simulink model "CSTFM_Pclass"  (Simulink 8.5)
settings: Solver=ode1  SolverMode=SingleTasking  StartTime=0.0  StopTime=200  FixedStep=25e-6  RelTol=1e-3
libraries: dspswit3 x1
settings Model: Creator=Administrator  LastModifiedBy=Administrator
settings DataIOCC: SignalLoggingSaveFormat=Dataset  SaveOutput=off  SaveTime=off
settings OptimizationCC: BlockReduction=off  OptimizeBlockIOStorage=off  BufferReuse=off  GlobalBufferReuse=off  ExpressionFolding=off  ExpressionDepthLimit=128  LocalBlockOutputs=off
settings DebuggingCC: UnderspecifiedInitializationDetection=Simplified  MergeDetectMultiDrivingBlocksExec=error  FcnCallInpInsideContextMsg=EnableAllAsError  StateNameClashWarn=none
settings GRTTargetCC: CombineOutputUpdateFcns=on  GRTInterface=off

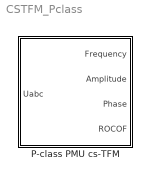
== system CSTFM_Pclass ==
  P-class PMU cs-TFM : Subsystem  SystemSampleTime=2e-4  VariantControl=variant3  mask{nominal_freq=50, T=0.06, Fs=5e3, Fr_50=50}
      mask prompts: nominal_freq "Norminal Frequency"; T "Window length (s)"; Fs "Sampling rate (Hz)"; Fr_50 "Data report rate (frames/s)"
      mask init:
      | %% // PUM initialization//
      | % the file is used to set basic paramters and creat initial matrix  
      | 
      | %% basic paramters
      | nominal_freq = 50;
      | T=0.06; %0.1;
      | TdF=10;
      | data_rate_50=1; %case: 1(10),2(25),3(50)
      | Fs=5e3;
      | P=11;
      | 
      | %% creat intial matrix
      | f0 = nominal_freq;
      | 
      | switch data_rate_50
      | case 1
      | Fr_50 = 10;
      | case 2
      | Fr_50 = 25;
      | case 3
      | Fr_50 = 50;
      | otherwise
      | display('Non contemplated data reporting rate')
      | end
      | 
      | Ts=1/Fs;
      | dF = 1/T;
      | M = round(T*Fs);
      | overlap=2*M/3;
      | kmax = round(f0*T);
      | k = (kmax-2):(kmax+7);
      | Wk = exp(-1i*2*pi*k./M);
      | NumIters=2;
      | Fr = Fr_50;
      | Tr = 1/Fr;
      | H = M*P;
      | 
      | h_axis = 0:Fs/H:Fs*(H-1)/H; % matrix h_aixs
      | 
      | D = zeros(M,H);%
      | for k = 0:M-1
      |     for h = 0:H-1
      |     esp = k - M*h/H;
      |     esp = esp*(M-1)/M;
      |     a = pi*(k-(h/H)*M);
      |     b = a/M;
      |     if b == pi || b == 0
      |         s = 1;
      |     else
      |         s = sin(a)/(M*sin(b));
      |     end
      |     D(k+1,h+1) = s*exp(-1i*pi*esp);
      |     end
      | end
      | 
      | D_funda=D(2:10, 31:37);%D(2:17,51:61);%
      | D_funda=D_funda'; 
      | inter_index=[8,11,14,17,51,54,57,60];%[12 17 23 28 83 89 94 100];
      | D_inter=D(2:10,inter_index);%D(2:17,inter_index);
      | D_inter=D_inter';
      | f_fund=h_axis(31:37);%h_axis(51:61);
      | % dft_rec=zeros(11,16);
      | % freq=(10:10:160);
      | % 
      | % for i=1:11
      | %     ff0=f_fund(i);
      | %     dft_rec(i,:) =(0.5*sinc((freq-ff0)*T)+0.25*sinc((freq-ff0-1/T)*T)+0.25*sinc((freq-ff0+1/T)*T))...
      | %     +  (0.5*sinc((-freq+ff0)*T)+0.25*sinc((-freq+ff0-1/T)*T)+0.25*sinc((-freq+ff0+1/T)*T));
      | % end
      | 
      | order = 2;
      | % M=3*M/5;
      | matrix_f=zeros(M,6,11);%
      | h=1;
      | Nh=M/2;
      | freq=(45:1:55);
      | for index=1:11
      |     omega1=2*pi*freq(index)/Fs;
      |     for i=0:M-1
      |         n = i - Nh;
      |         nc = 0;
      |         facts = factorial(2:-1:0);
      |         e = exp(1j*n*h*omega1);
      |         matrix_f(i+1,nc+1:nc+2*order+2,index) = [(((n*Ts).^...
      |             (order:-1:0)).*e)./facts, (((n*Ts).^...
      |             (0:1:order)).*e')./fliplr(facts)];
      |     end
      | end
      | 
      | matrix_har2=zeros(M,6,11); %
      | freq=2*(45:1:55);
      | for index=1:11
      |     omega1=2*pi*freq(index)/Fs;
      |     for i=0:M-1
      |         n = i - Nh;
      |         nc = 0;
      |         facts = factorial(2:-1:0);
      |         e = exp(1j*n*h*omega1);
      |         matrix_har2(i+1,nc+1:nc+2*order+2,index) = [(((n*Ts).^...
      |             (order:-1:0)).*e)./facts, (((n*Ts).^...
      |             (0:1:order)).*e')./fliplr(facts)];
      |     end
      | end
      | 
      | matrix_har3=zeros(M,6,11);%
      | freq=3*(45:1:55);
      | for index=1:11
      |     omega1=2*pi*freq(index)/Fs;
      |     for i=0:M-1
      |         n = i - Nh;
      |         nc = 0;
      |         facts = factorial(2:-1:0);
      |         e = exp(1j*n*h*omega1);
      |         matrix_har3(i+1,nc+1:nc+2*order+2,index) = [(((n*Ts).^...
      |             (order:-1:0)).*e)./facts, (((n*Ts).^...
      |             (0:1:order)).*e')./fliplr(facts)];
      |     end
      | end
      | 
      | % M = round(T*Fs);
      | clear D
      mask TypeOptions Fr_50: 10 | 25 | 50

== system CSTFM_Pclass/P-class PMU cs-TFM ==
  Uabc : Inport
  Buffer : Buffer  N=M  V=overlap  TreatMby1Signals=One channel
  Demux : Demux  Outputs=3
  Rate Transition : RateTransition  OutPortSampleTime=2e-4
  Subsystem : Subsystem  TreatAsAtomicUnit=on  SystemSampleTime=Ts*(M-overlap)
  Terminator : Terminator
  Terminator1 : Terminator
  msdft Hanning : Subsystem  TreatAsAtomicUnit=on  SystemSampleTime=2e-4
  Frequency : Outport
  Amplitude : Outport  Port=2
  Phase : Outport  Port=3
  ROCOF : Outport  Port=4
  wires:
  Uabc/1 -> Demux/1
  Rate Transition/1 -> Buffer/1
  msdft Hanning/1(DFT) -> Subsystem/2(A)
  Subsystem/4(RoCoF) -> ROCOF/1
  Subsystem/3(frequency) -> Frequency/1
  Subsystem/2(phase_estimated) -> Phase/1
  Subsystem/1(Amplitude) -> Amplitude/1
  Buffer/1 -> Subsystem/1(buffer_a)
  Demux/3 -> Terminator1/1
  Demux/2 -> Terminator/1
  Demux/1 -> msdft Hanning/1(signal), Rate Transition/1  "Ua"

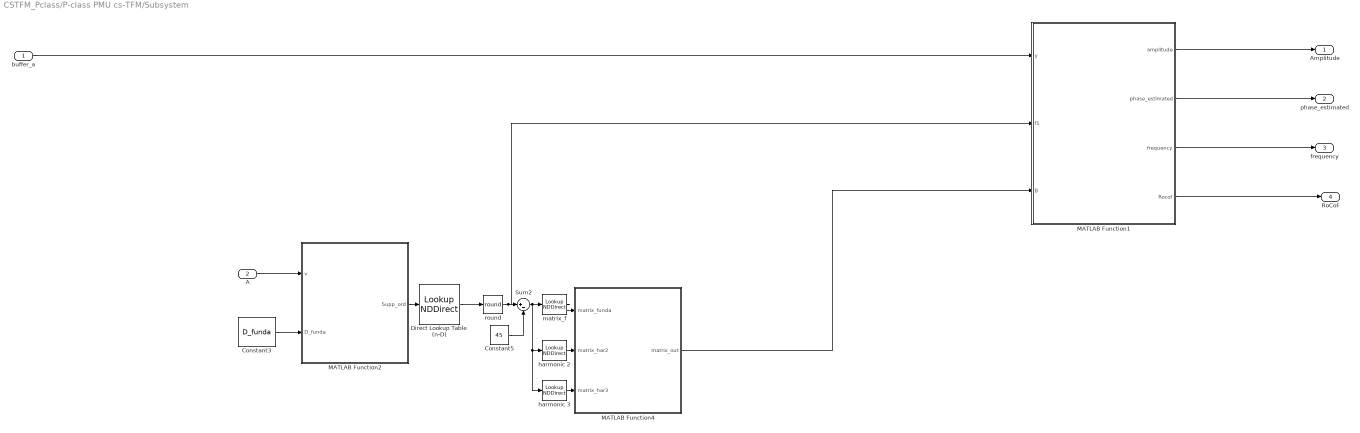
== system CSTFM_Pclass/P-class PMU cs-TFM/Subsystem ==
  buffer_a : Inport
  A : Inport  Port=2
  Constant3 : Constant  Value=D_funda
  Constant5 : Constant  Value=45
  Direct Lookup Table (n-D) : LookupNDDirect  NumberOfTableDimensions=1  Table=h_axis
  MATLAB Function1 : MATLAB Function  RequirementInfo={} %GIDa_f55fb0f0_c66f_4964_a101_9f74e0196493  SystemSampleTime=Ts*(M-overlap)
  MATLAB Function2 : MATLAB Function  SystemSampleTime=Ts*(M-overlap)
  MATLAB Function4 : MATLAB Function  RequirementInfo={} %GIDa_9de8f8bb_0410_4add_86be_2b397df83b55  SystemSampleTime=Ts*(M-overlap)
  Sum2 : Sum  Inputs=|+-
  harmonic 2 : LookupNDDirect  NumberOfTableDimensions=3  InputsSelectThisObjectFromTable=2-D Matrix  Table=matrix_har2
  "harmonic 3 " : LookupNDDirect  NumberOfTableDimensions=3  InputsSelectThisObjectFromTable=2-D Matrix  Table=matrix_har3
  matrix_f : LookupNDDirect  NumberOfTableDimensions=3  InputsSelectThisObjectFromTable=2-D Matrix  Table=matrix_f
  round : Rounding  Operator=round
  Amplitude : Outport
  phase_estimated : Outport  Port=2
  frequency : Outport  Port=3
  RoCoF : Outport  Port=4
  wires:
  Direct Lookup Table (n-D)/1 -> round/1
  MATLAB Function1/4(Rocof) -> RoCoF/1
  buffer_a/1 -> MATLAB Function1/1(y)
  round/1 -> Sum2/1, MATLAB Function1/2(f1)
  Constant3/1 -> MATLAB Function2/2(D_funda)
  MATLAB Function2/1(Supp_ord) -> Direct Lookup Table (n-D)/1
  A/1 -> MATLAB Function2/1(v)
  matrix_f/1 -> MATLAB Function4/1(matrix_funda)
  Sum2/1 -> "harmonic 3 "/1, harmonic 2/1, matrix_f/1
  Constant5/1 -> Sum2/2
  harmonic 2/1 -> MATLAB Function4/2(matrix_har2)
  "harmonic 3 "/1 -> MATLAB Function4/3(matrix_har3)
  MATLAB Function4/1(matrix_out) -> MATLAB Function1/3(B)
  MATLAB Function1/1(amplitude) -> Amplitude/1
  MATLAB Function1/2(phase_estimated) -> phase_estimated/1
  MATLAB Function1/3(frequency) -> frequency/1

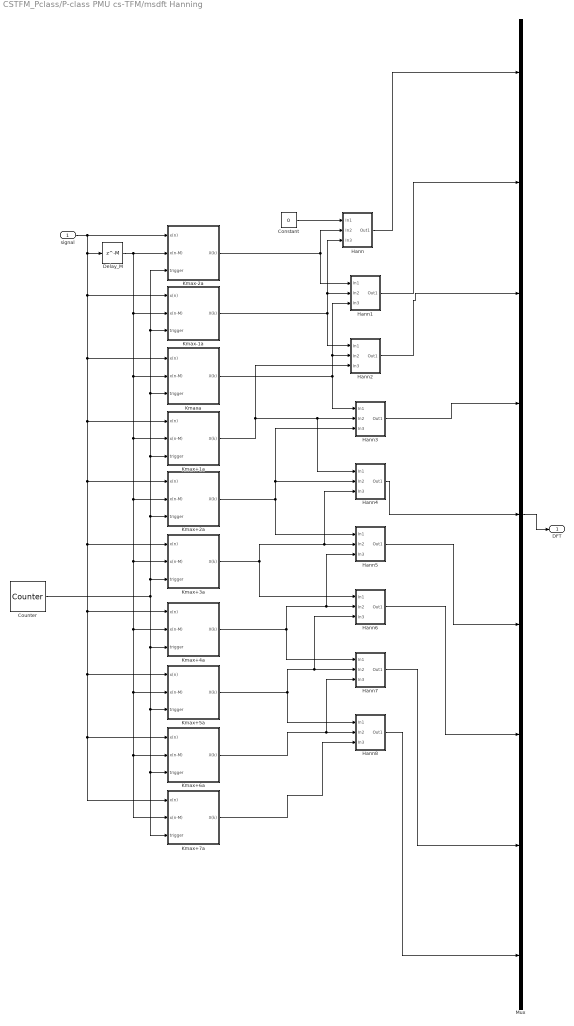
== system CSTFM_Pclass/P-class PMU cs-TFM/msdft Hanning ==
  signal : Inport
  Constant : Constant  Value=0
  Counter : dspswit3/Counter  Direction=Up  CountEvent=Free running  CounterSize=User defined  MaxCount=M-1  InitialCount=1  Output=Hit  HitValue=0  ResetInput=off  SamplesPerFrame=1  Ts=Ts  CntDtype=double  HitDtype=Logical
  Delay_M : Delay  DelayLength=M
  Hann : Subsystem
  Hann1 : Subsystem
  Hann2 : Subsystem
  Hann3 : Subsystem
  Hann4 : Subsystem
  Hann5 : Subsystem
  Hann6 : Subsystem
  Hann7 : Subsystem
  Hann8 : Subsystem
  Kmax+1a : Subsystem
  Kmax+2a : Subsystem
  Kmax+3a : Subsystem
  Kmax+4a : Subsystem
  Kmax+5a : Subsystem
  Kmax+6a : Subsystem
  Kmax+7a : Subsystem
  Kmax-1a : Subsystem
  Kmax-2a : Subsystem
  Kmaxa : Subsystem
  Mux : Mux  Inputs=9
  DFT : Outport
  wires:
  Counter/1 -> Kmax+5a/3(trigger), Kmax+7a/3(trigger), Kmax+6a/3(trigger), Kmax+4a/3(trigger), Kmax+2a/3(trigger), Kmax+1a/3(trigger), Kmax-1a/3(trigger), Kmax-2a/3(trigger), Kmaxa/3(trigger), Kmax+3a/3(trigger)
  Kmax-2a/1(X(k)) -> Hann/2(In2), Hann1/1(In1)
  Kmax-1a/1(X(k)) -> Hann2/1(In1), Hann1/2(In2), Hann/3(In3)
  Kmaxa/1(X(k)) -> Hann3/1(In1), Hann2/2(In2), Hann1/3(In3)
  Kmax+1a/1(X(k)) -> Hann2/3(In3), Hann4/1(In1), Hann3/2(In2)
  Kmax+2a/1(X(k)) -> Hann4/2(In2), Hann3/3(In3), Hann5/1(In1)
  Kmax+4a/1(X(k)) -> Hann7/1(In1), Hann5/3(In3), Hann6/2(In2)
  Kmax+6a/1(X(k)) -> Hann7/3(In3), Hann8/2(In2)
  Mux/1 -> DFT/1
  signal/1 -> Kmax+7a/1(x(n)), Kmax+6a/1(x(n)), Kmax+5a/1(x(n)), Kmax+4a/1(x(n)), Kmax+3a/1(x(n)), Kmax+2a/1(x(n)), Kmax+1a/1(x(n)), Kmaxa/1(x(n)), Kmax-1a/1(x(n)), Delay_M/1, Kmax-2a/1(x(n))
  Delay_M/1 -> Kmax+5a/2(x(n-M)), Kmax+7a/2(x(n-M)), Kmax+6a/2(x(n-M)), Kmax+4a/2(x(n-M)), Kmax+3a/2(x(n-M)), Kmax+2a/2(x(n-M)), Kmax+1a/2(x(n-M)), Kmaxa/2(x(n-M)), Kmax-1a/2(x(n-M)), Kmax-2a/2(x(n-M))
  Hann/1(Out1) -> Mux/1
  Constant/1 -> Hann/1(In1)
  Hann1/1(Out1) -> Mux/2
  Hann2/1(Out1) -> Mux/3
  Hann3/1(Out1) -> Mux/4
  Hann4/1(Out1) -> Mux/5
  Hann5/1(Out1) -> Mux/6
  Hann6/1(Out1) -> Mux/7
  Hann7/1(Out1) -> Mux/8
  Hann8/1(Out1) -> Mux/9
  Kmax+7a/1(X(k)) -> Hann8/3(In3)
  Kmax+5a/1(X(k)) -> Hann8/1(In1), Hann6/3(In3), Hann7/2(In2)
  Kmax+3a/1(X(k)) -> Hann4/3(In3), Hann5/2(In2), Hann6/1(In1)

== system CSTFM_Pclass/P-class PMU cs-TFM/msdft Hanning/Hann ==
  In1 : Inport
  In2 : Inport  Port=2
  In3 : Inport  Port=3
  Gain : Gain  Gain=-0.25
  Gain1 : Gain  Gain=0.5
  Gain2 : Gain  Gain=-0.25
  Sum : Sum  Inputs=|+++
  Out1 : Outport
  wires:
  Sum/1 -> Out1/1
  In3/1 -> Gain2/1
  In1/1 -> Gain/1
  In2/1 -> Gain1/1
  Gain2/1 -> Sum/3
  Gain1/1 -> Sum/2
  Gain/1 -> Sum/1

== system CSTFM_Pclass/P-class PMU cs-TFM/msdft Hanning/Hann1 ==
  In1 : Inport
  In2 : Inport  Port=2
  In3 : Inport  Port=3
  Gain : Gain  Gain=-0.25
  Gain1 : Gain  Gain=0.5
  Gain2 : Gain  Gain=-0.25
  Sum : Sum  Inputs=|+++
  Out1 : Outport
  wires:
  Sum/1 -> Out1/1
  In3/1 -> Gain2/1
  In1/1 -> Gain/1
  In2/1 -> Gain1/1
  Gain2/1 -> Sum/3
  Gain1/1 -> Sum/2
  Gain/1 -> Sum/1

== system CSTFM_Pclass/P-class PMU cs-TFM/msdft Hanning/Hann2 ==
  In1 : Inport
  In2 : Inport  Port=2
  In3 : Inport  Port=3
  Gain : Gain  Gain=-0.25
  Gain1 : Gain  Gain=0.5
  Gain2 : Gain  Gain=-0.25
  Sum : Sum  Inputs=|+++
  Out1 : Outport
  wires:
  Sum/1 -> Out1/1
  In3/1 -> Gain2/1
  In1/1 -> Gain/1
  In2/1 -> Gain1/1
  Gain2/1 -> Sum/3
  Gain1/1 -> Sum/2
  Gain/1 -> Sum/1

== system CSTFM_Pclass/P-class PMU cs-TFM/msdft Hanning/Hann3 ==
  In1 : Inport
  In2 : Inport  Port=2
  In3 : Inport  Port=3
  Gain : Gain  Gain=-0.25
  Gain1 : Gain  Gain=0.5
  Gain2 : Gain  Gain=-0.25
  Sum : Sum  Inputs=|+++
  Out1 : Outport
  wires:
  Sum/1 -> Out1/1
  In3/1 -> Gain2/1
  In1/1 -> Gain/1
  In2/1 -> Gain1/1
  Gain2/1 -> Sum/3
  Gain1/1 -> Sum/2
  Gain/1 -> Sum/1

== system CSTFM_Pclass/P-class PMU cs-TFM/msdft Hanning/Hann4 ==
  In1 : Inport
  In2 : Inport  Port=2
  In3 : Inport  Port=3
  Gain : Gain  Gain=-0.25
  Gain1 : Gain  Gain=0.5
  Gain2 : Gain  Gain=-0.25
  Sum : Sum  Inputs=|+++
  Out1 : Outport
  wires:
  Sum/1 -> Out1/1
  In3/1 -> Gain2/1
  In1/1 -> Gain/1
  In2/1 -> Gain1/1
  Gain2/1 -> Sum/3
  Gain1/1 -> Sum/2
  Gain/1 -> Sum/1

== system CSTFM_Pclass/P-class PMU cs-TFM/msdft Hanning/Hann5 ==
  In1 : Inport
  In2 : Inport  Port=2
  In3 : Inport  Port=3
  Gain : Gain  Gain=-0.25
  Gain1 : Gain  Gain=0.5
  Gain2 : Gain  Gain=-0.25
  Sum : Sum  Inputs=|+++
  Out1 : Outport
  wires:
  Sum/1 -> Out1/1
  In3/1 -> Gain2/1
  In1/1 -> Gain/1
  In2/1 -> Gain1/1
  Gain2/1 -> Sum/3
  Gain1/1 -> Sum/2
  Gain/1 -> Sum/1

== system CSTFM_Pclass/P-class PMU cs-TFM/msdft Hanning/Hann6 ==
  In1 : Inport
  In2 : Inport  Port=2
  In3 : Inport  Port=3
  Gain : Gain  Gain=-0.25
  Gain1 : Gain  Gain=0.5
  Gain2 : Gain  Gain=-0.25
  Sum : Sum  Inputs=|+++
  Out1 : Outport
  wires:
  Sum/1 -> Out1/1
  In3/1 -> Gain2/1
  In1/1 -> Gain/1
  In2/1 -> Gain1/1
  Gain2/1 -> Sum/3
  Gain1/1 -> Sum/2
  Gain/1 -> Sum/1

== system CSTFM_Pclass/P-class PMU cs-TFM/msdft Hanning/Hann7 ==
  In1 : Inport
  In2 : Inport  Port=2
  In3 : Inport  Port=3
  Gain : Gain  Gain=-0.25
  Gain1 : Gain  Gain=0.5
  Gain2 : Gain  Gain=-0.25
  Sum : Sum  Inputs=|+++
  Out1 : Outport
  wires:
  Sum/1 -> Out1/1
  In3/1 -> Gain2/1
  In1/1 -> Gain/1
  In2/1 -> Gain1/1
  Gain2/1 -> Sum/3
  Gain1/1 -> Sum/2
  Gain/1 -> Sum/1

== system CSTFM_Pclass/P-class PMU cs-TFM/msdft Hanning/Hann8 ==
  In1 : Inport
  In2 : Inport  Port=2
  In3 : Inport  Port=3
  Gain : Gain  Gain=-0.25
  Gain1 : Gain  Gain=0.5
  Gain2 : Gain  Gain=-0.25
  Sum : Sum  Inputs=|+++
  Out1 : Outport
  wires:
  Sum/1 -> Out1/1
  In3/1 -> Gain2/1
  In1/1 -> Gain/1
  In2/1 -> Gain1/1
  Gain2/1 -> Sum/3
  Gain1/1 -> Sum/2
  Gain/1 -> Sum/1

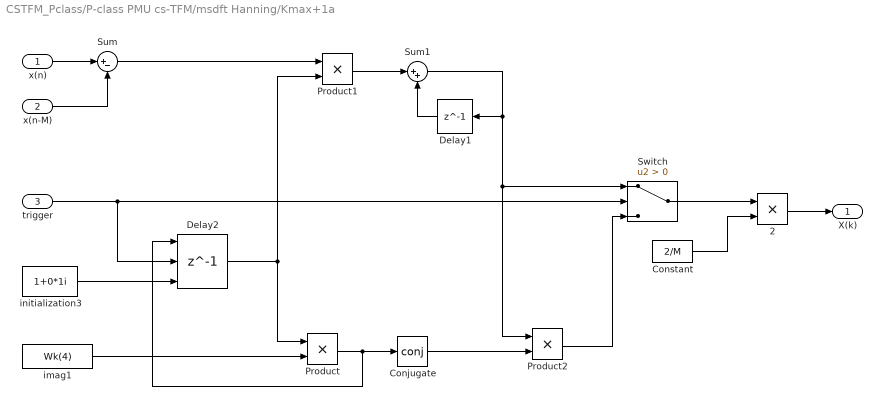
== system CSTFM_Pclass/P-class PMU cs-TFM/msdft Hanning/Kmax+1a ==
  x(n) : Inport
  x(n-M) : Inport  Port=2
  trigger : Inport  Port=3
  2 : Product  RndMeth=Zero
  Conjugate : Math  Operator=conj  SaturateOnIntegerOverflow=on
  Constant : Constant  Value=2/M
  Delay1 : Delay  DelayLength=1
  Delay2 : Delay  DelayLength=1  InitialConditionSource=Input port  ExternalReset=Falling
      settings: InputPortMap=u0,r5,p4
  Product : Product  RndMeth=Zero
  Product1 : Product  RndMeth=Zero
  Product2 : Product  RndMeth=Zero
  Sum : Sum  Inputs=|+-
  Sum1 : Sum  Inputs=|++
  Switch : Switch  Criteria=u2 > Threshold
  imag1 : Constant  Value=Wk(4)
  initialization3 : Constant  Value=1+0*1i
  X(k) : Outport
  wires:
  Switch/1 -> 2/1
  Product2/1 -> Switch/3
  Conjugate/1 -> Product2/2
  Product/1 -> Conjugate/1, Delay2/1
  imag1/1 -> Product/2
  initialization3/1 -> Delay2/3
  Delay2/1 -> Product/1, Product1/2
  trigger/1 -> Switch/2, Delay2/2
  2/1 -> X(k)/1
  Constant/1 -> 2/2
  Sum/1 -> Product1/1
  x(n-M)/1 -> Sum/2
  x(n)/1 -> Sum/1
  Delay1/1 -> Sum1/2
  Sum1/1 -> Product2/1, Switch/1, Delay1/1
  Product1/1 -> Sum1/1

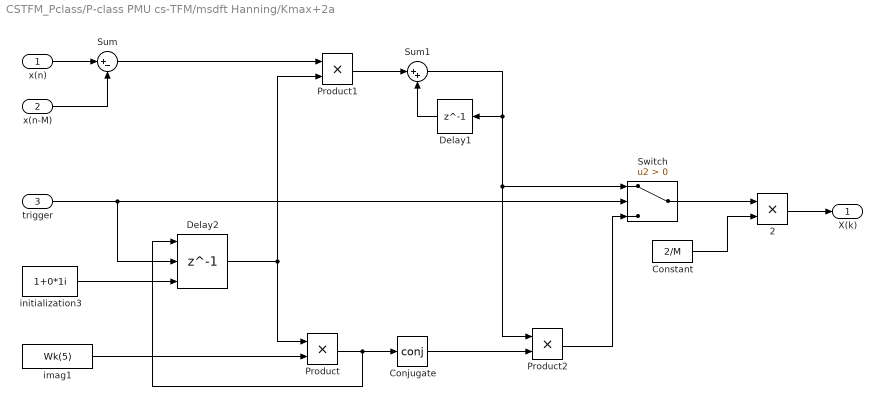
== system CSTFM_Pclass/P-class PMU cs-TFM/msdft Hanning/Kmax+2a ==
  x(n) : Inport
  x(n-M) : Inport  Port=2
  trigger : Inport  Port=3
  2 : Product  RndMeth=Zero
  Conjugate : Math  Operator=conj  SaturateOnIntegerOverflow=on
  Constant : Constant  Value=2/M
  Delay1 : Delay  DelayLength=1
  Delay2 : Delay  DelayLength=1  InitialConditionSource=Input port  ExternalReset=Falling
      settings: InputPortMap=u0,r5,p4
  Product : Product  RndMeth=Zero
  Product1 : Product  RndMeth=Zero
  Product2 : Product  RndMeth=Zero
  Sum : Sum  Inputs=|+-
  Sum1 : Sum  Inputs=|++
  Switch : Switch  Criteria=u2 > Threshold
  imag1 : Constant  Value=Wk(5)
  initialization3 : Constant  Value=1+0*1i
  X(k) : Outport
  wires:
  Switch/1 -> 2/1
  Product2/1 -> Switch/3
  Conjugate/1 -> Product2/2
  Product/1 -> Conjugate/1, Delay2/1
  imag1/1 -> Product/2
  initialization3/1 -> Delay2/3
  Delay2/1 -> Product/1, Product1/2
  trigger/1 -> Switch/2, Delay2/2
  2/1 -> X(k)/1
  Constant/1 -> 2/2
  Sum/1 -> Product1/1
  x(n-M)/1 -> Sum/2
  x(n)/1 -> Sum/1
  Delay1/1 -> Sum1/2
  Sum1/1 -> Product2/1, Switch/1, Delay1/1
  Product1/1 -> Sum1/1

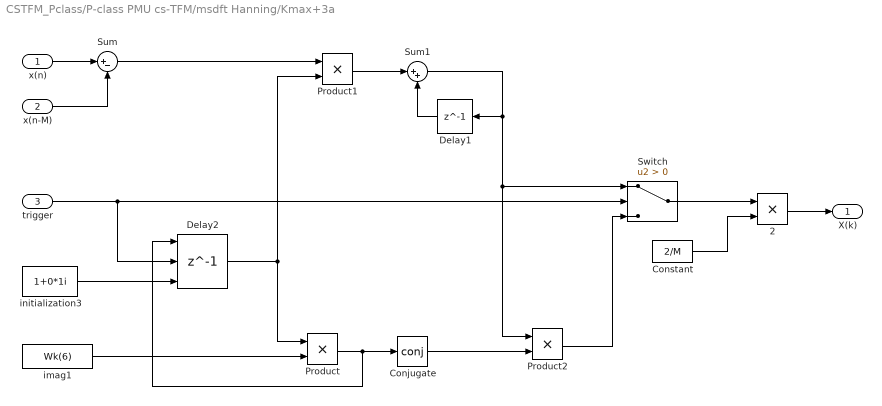
== system CSTFM_Pclass/P-class PMU cs-TFM/msdft Hanning/Kmax+3a ==
  x(n) : Inport
  x(n-M) : Inport  Port=2
  trigger : Inport  Port=3
  2 : Product  RndMeth=Zero
  Conjugate : Math  Operator=conj  SaturateOnIntegerOverflow=on
  Constant : Constant  Value=2/M
  Delay1 : Delay  DelayLength=1
  Delay2 : Delay  DelayLength=1  InitialConditionSource=Input port  ExternalReset=Falling
      settings: InputPortMap=u0,r5,p4
  Product : Product  RndMeth=Zero
  Product1 : Product  RndMeth=Zero
  Product2 : Product  RndMeth=Zero
  Sum : Sum  Inputs=|+-
  Sum1 : Sum  Inputs=|++
  Switch : Switch  Criteria=u2 > Threshold
  imag1 : Constant  Value=Wk(6)
  initialization3 : Constant  Value=1+0*1i
  X(k) : Outport
  wires:
  Switch/1 -> 2/1
  Product2/1 -> Switch/3
  Conjugate/1 -> Product2/2
  Product/1 -> Conjugate/1, Delay2/1
  imag1/1 -> Product/2
  initialization3/1 -> Delay2/3
  Delay2/1 -> Product/1, Product1/2
  trigger/1 -> Switch/2, Delay2/2
  2/1 -> X(k)/1
  Constant/1 -> 2/2
  Sum/1 -> Product1/1
  x(n-M)/1 -> Sum/2
  x(n)/1 -> Sum/1
  Delay1/1 -> Sum1/2
  Sum1/1 -> Product2/1, Switch/1, Delay1/1
  Product1/1 -> Sum1/1

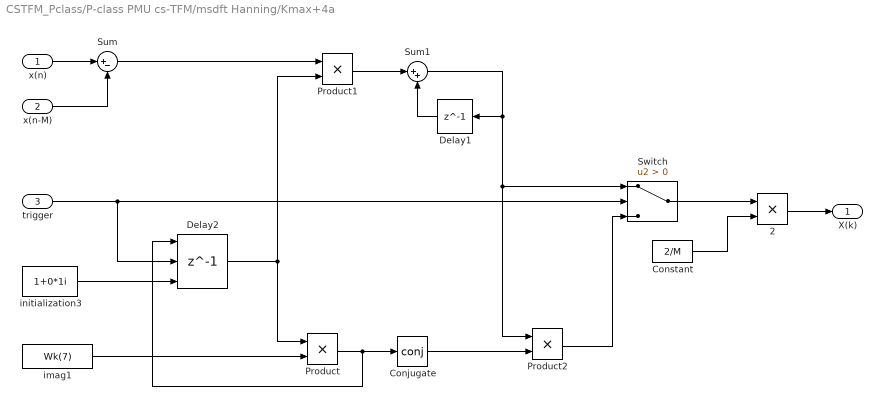
== system CSTFM_Pclass/P-class PMU cs-TFM/msdft Hanning/Kmax+4a ==
  x(n) : Inport
  x(n-M) : Inport  Port=2
  trigger : Inport  Port=3
  2 : Product  RndMeth=Zero
  Conjugate : Math  Operator=conj  SaturateOnIntegerOverflow=on
  Constant : Constant  Value=2/M
  Delay1 : Delay  DelayLength=1
  Delay2 : Delay  DelayLength=1  InitialConditionSource=Input port  ExternalReset=Falling
      settings: InputPortMap=u0,r5,p4
  Product : Product  RndMeth=Zero
  Product1 : Product  RndMeth=Zero
  Product2 : Product  RndMeth=Zero
  Sum : Sum  Inputs=|+-
  Sum1 : Sum  Inputs=|++
  Switch : Switch  Criteria=u2 > Threshold
  imag1 : Constant  Value=Wk(7)
  initialization3 : Constant  Value=1+0*1i
  X(k) : Outport
  wires:
  Switch/1 -> 2/1
  Product2/1 -> Switch/3
  Conjugate/1 -> Product2/2
  Product/1 -> Conjugate/1, Delay2/1
  imag1/1 -> Product/2
  initialization3/1 -> Delay2/3
  Delay2/1 -> Product/1, Product1/2
  trigger/1 -> Switch/2, Delay2/2
  2/1 -> X(k)/1
  Constant/1 -> 2/2
  Sum/1 -> Product1/1
  x(n-M)/1 -> Sum/2
  x(n)/1 -> Sum/1
  Delay1/1 -> Sum1/2
  Sum1/1 -> Product2/1, Switch/1, Delay1/1
  Product1/1 -> Sum1/1

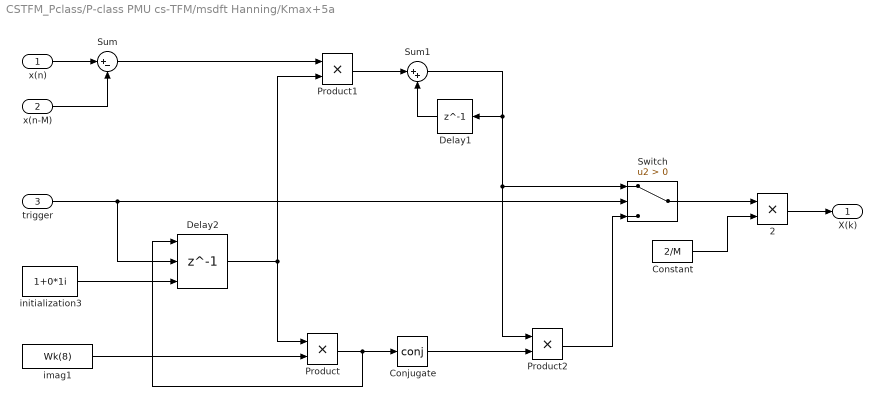
== system CSTFM_Pclass/P-class PMU cs-TFM/msdft Hanning/Kmax+5a ==
  x(n) : Inport
  x(n-M) : Inport  Port=2
  trigger : Inport  Port=3
  2 : Product  RndMeth=Zero
  Conjugate : Math  Operator=conj  SaturateOnIntegerOverflow=on
  Constant : Constant  Value=2/M
  Delay1 : Delay  DelayLength=1
  Delay2 : Delay  DelayLength=1  InitialConditionSource=Input port  ExternalReset=Falling
      settings: InputPortMap=u0,r5,p4
  Product : Product  RndMeth=Zero
  Product1 : Product  RndMeth=Zero
  Product2 : Product  RndMeth=Zero
  Sum : Sum  Inputs=|+-
  Sum1 : Sum  Inputs=|++
  Switch : Switch  Criteria=u2 > Threshold
  imag1 : Constant  Value=Wk(8)
  initialization3 : Constant  Value=1+0*1i
  X(k) : Outport
  wires:
  Switch/1 -> 2/1
  Product2/1 -> Switch/3
  Conjugate/1 -> Product2/2
  Product/1 -> Conjugate/1, Delay2/1
  imag1/1 -> Product/2
  initialization3/1 -> Delay2/3
  Delay2/1 -> Product/1, Product1/2
  trigger/1 -> Switch/2, Delay2/2
  2/1 -> X(k)/1
  Constant/1 -> 2/2
  Sum/1 -> Product1/1
  x(n-M)/1 -> Sum/2
  x(n)/1 -> Sum/1
  Delay1/1 -> Sum1/2
  Sum1/1 -> Product2/1, Switch/1, Delay1/1
  Product1/1 -> Sum1/1

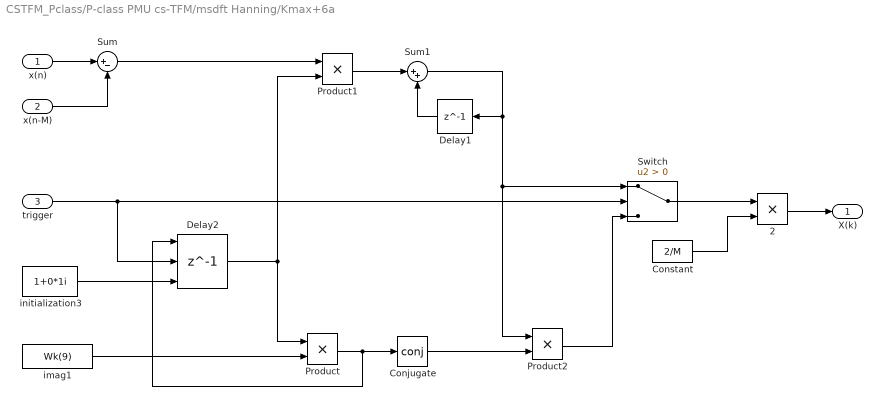
== system CSTFM_Pclass/P-class PMU cs-TFM/msdft Hanning/Kmax+6a ==
  x(n) : Inport
  x(n-M) : Inport  Port=2
  trigger : Inport  Port=3
  2 : Product  RndMeth=Zero
  Conjugate : Math  Operator=conj  SaturateOnIntegerOverflow=on
  Constant : Constant  Value=2/M
  Delay1 : Delay  DelayLength=1
  Delay2 : Delay  DelayLength=1  InitialConditionSource=Input port  ExternalReset=Falling
      settings: InputPortMap=u0,r5,p4
  Product : Product  RndMeth=Zero
  Product1 : Product  RndMeth=Zero
  Product2 : Product  RndMeth=Zero
  Sum : Sum  Inputs=|+-
  Sum1 : Sum  Inputs=|++
  Switch : Switch  Criteria=u2 > Threshold
  imag1 : Constant  Value=Wk(9)
  initialization3 : Constant  Value=1+0*1i
  X(k) : Outport
  wires:
  Switch/1 -> 2/1
  Product2/1 -> Switch/3
  Conjugate/1 -> Product2/2
  Product/1 -> Conjugate/1, Delay2/1
  imag1/1 -> Product/2
  initialization3/1 -> Delay2/3
  Delay2/1 -> Product/1, Product1/2
  trigger/1 -> Switch/2, Delay2/2
  2/1 -> X(k)/1
  Constant/1 -> 2/2
  Sum/1 -> Product1/1
  x(n-M)/1 -> Sum/2
  x(n)/1 -> Sum/1
  Delay1/1 -> Sum1/2
  Sum1/1 -> Product2/1, Switch/1, Delay1/1
  Product1/1 -> Sum1/1

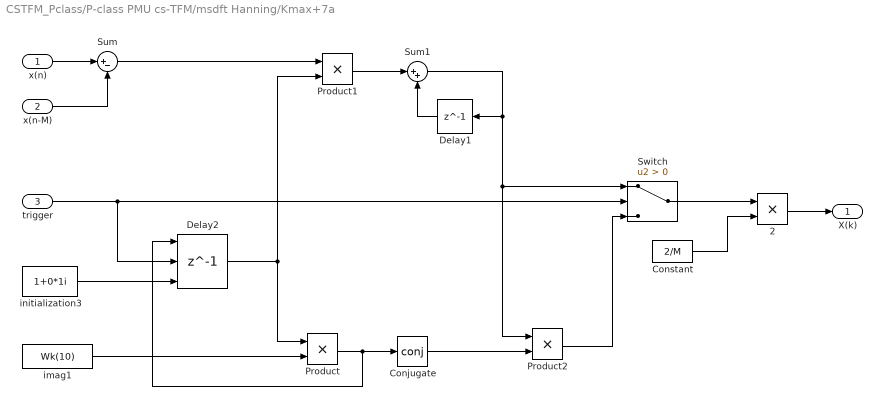
== system CSTFM_Pclass/P-class PMU cs-TFM/msdft Hanning/Kmax+7a ==
  x(n) : Inport
  x(n-M) : Inport  Port=2
  trigger : Inport  Port=3
  2 : Product  RndMeth=Zero
  Conjugate : Math  Operator=conj  SaturateOnIntegerOverflow=on
  Constant : Constant  Value=2/M
  Delay1 : Delay  DelayLength=1
  Delay2 : Delay  DelayLength=1  InitialConditionSource=Input port  ExternalReset=Falling
      settings: InputPortMap=u0,r5,p4
  Product : Product  RndMeth=Zero
  Product1 : Product  RndMeth=Zero
  Product2 : Product  RndMeth=Zero
  Sum : Sum  Inputs=|+-
  Sum1 : Sum  Inputs=|++
  Switch : Switch  Criteria=u2 > Threshold
  imag1 : Constant  Value=Wk(10)
  initialization3 : Constant  Value=1+0*1i
  X(k) : Outport
  wires:
  Switch/1 -> 2/1
  Product2/1 -> Switch/3
  Conjugate/1 -> Product2/2
  Product/1 -> Conjugate/1, Delay2/1
  imag1/1 -> Product/2
  initialization3/1 -> Delay2/3
  Delay2/1 -> Product/1, Product1/2
  trigger/1 -> Switch/2, Delay2/2
  2/1 -> X(k)/1
  Constant/1 -> 2/2
  Sum/1 -> Product1/1
  x(n-M)/1 -> Sum/2
  x(n)/1 -> Sum/1
  Delay1/1 -> Sum1/2
  Sum1/1 -> Product2/1, Switch/1, Delay1/1
  Product1/1 -> Sum1/1

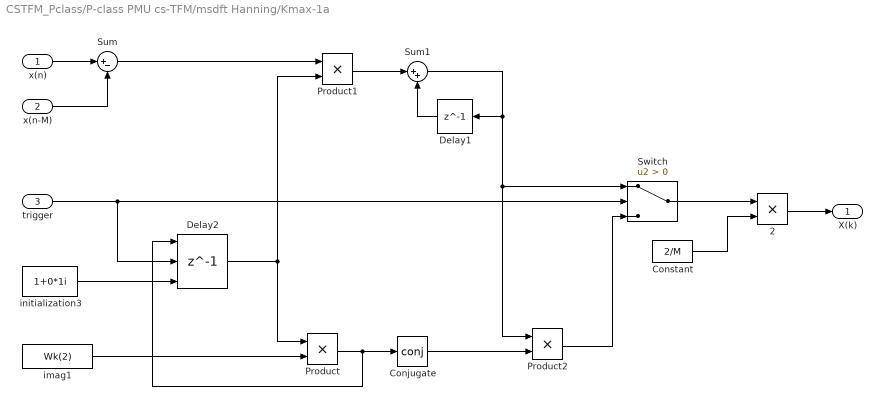
== system CSTFM_Pclass/P-class PMU cs-TFM/msdft Hanning/Kmax-1a ==
  x(n) : Inport
  x(n-M) : Inport  Port=2
  trigger : Inport  Port=3
  2 : Product  RndMeth=Zero
  Conjugate : Math  Operator=conj  SaturateOnIntegerOverflow=on
  Constant : Constant  Value=2/M
  Delay1 : Delay  DelayLength=1
  Delay2 : Delay  DelayLength=1  InitialConditionSource=Input port  ExternalReset=Falling
      settings: InputPortMap=u0,r5,p4
  Product : Product  RndMeth=Zero
  Product1 : Product  RndMeth=Zero
  Product2 : Product  RndMeth=Zero
  Sum : Sum  Inputs=|+-
  Sum1 : Sum  Inputs=|++
  Switch : Switch  Criteria=u2 > Threshold
  imag1 : Constant  Value=Wk(2)
  initialization3 : Constant  Value=1+0*1i
  X(k) : Outport
  wires:
  Switch/1 -> 2/1
  Product2/1 -> Switch/3
  Conjugate/1 -> Product2/2
  Product/1 -> Conjugate/1, Delay2/1
  imag1/1 -> Product/2
  initialization3/1 -> Delay2/3
  Delay2/1 -> Product/1, Product1/2
  trigger/1 -> Switch/2, Delay2/2
  2/1 -> X(k)/1
  Constant/1 -> 2/2
  Sum/1 -> Product1/1
  x(n-M)/1 -> Sum/2
  x(n)/1 -> Sum/1
  Delay1/1 -> Sum1/2
  Sum1/1 -> Product2/1, Switch/1, Delay1/1
  Product1/1 -> Sum1/1

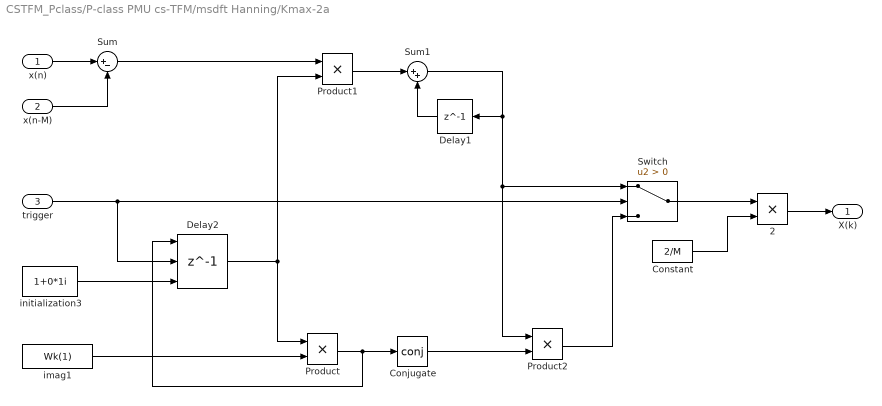
== system CSTFM_Pclass/P-class PMU cs-TFM/msdft Hanning/Kmax-2a ==
  x(n) : Inport
  x(n-M) : Inport  Port=2
  trigger : Inport  Port=3
  2 : Product  RndMeth=Zero
  Conjugate : Math  Operator=conj  SaturateOnIntegerOverflow=on
  Constant : Constant  Value=2/M
  Delay1 : Delay  DelayLength=1
  Delay2 : Delay  DelayLength=1  InitialConditionSource=Input port  ExternalReset=Falling
      settings: InputPortMap=u0,r5,p4
  Product : Product  RndMeth=Zero
  Product1 : Product  RndMeth=Zero
  Product2 : Product  RndMeth=Zero
  Sum : Sum  Inputs=|+-
  Sum1 : Sum  Inputs=|++
  Switch : Switch  Criteria=u2 > Threshold
  imag1 : Constant  Value=Wk(1)
  initialization3 : Constant  Value=1+0*1i
  X(k) : Outport
  wires:
  Switch/1 -> 2/1
  Product2/1 -> Switch/3
  Conjugate/1 -> Product2/2
  Product/1 -> Conjugate/1, Delay2/1
  imag1/1 -> Product/2
  initialization3/1 -> Delay2/3
  Delay2/1 -> Product/1, Product1/2
  trigger/1 -> Switch/2, Delay2/2
  2/1 -> X(k)/1
  Constant/1 -> 2/2
  Sum/1 -> Product1/1
  x(n-M)/1 -> Sum/2
  x(n)/1 -> Sum/1
  Delay1/1 -> Sum1/2
  Sum1/1 -> Product2/1, Switch/1, Delay1/1
  Product1/1 -> Sum1/1

== system CSTFM_Pclass/P-class PMU cs-TFM/msdft Hanning/Kmaxa ==
  x(n) : Inport
  x(n-M) : Inport  Port=2
  trigger : Inport  Port=3
  2 : Product  RndMeth=Zero
  Conjugate : Math  Operator=conj  SaturateOnIntegerOverflow=on
  Constant : Constant  Value=2/M
  Delay1 : Delay  DelayLength=1
  Delay2 : Delay  DelayLength=1  InitialConditionSource=Input port  ExternalReset=Falling
      settings: InputPortMap=u0,r5,p4
  Product : Product  RndMeth=Zero
  Product1 : Product  RndMeth=Zero
  Product2 : Product  RndMeth=Zero
  Sum : Sum  Inputs=|+-
  Sum1 : Sum  Inputs=|++
  Switch : Switch  Criteria=u2 > Threshold
  imag1 : Constant  Value=Wk(3)
  initialization3 : Constant  Value=1+0*1i
  X(k) : Outport
  wires:
  Switch/1 -> 2/1
  Product2/1 -> Switch/3
  Conjugate/1 -> Product2/2
  Product/1 -> Conjugate/1, Delay2/1
  imag1/1 -> Product/2
  initialization3/1 -> Delay2/3
  Delay2/1 -> Product/1, Product1/2
  trigger/1 -> Switch/2, Delay2/2
  2/1 -> X(k)/1
  Constant/1 -> 2/2
  Sum/1 -> Product1/1
  x(n-M)/1 -> Sum/2
  x(n)/1 -> Sum/1
  Delay1/1 -> Sum1/2
  Sum1/1 -> Product2/1, Switch/1, Delay1/1
  Product1/1 -> Sum1/1

== matlab function P-class PMU cs-TFM/Subsystem/MATLAB Function1 ==
  data: y input double; f1 input double; amplitude output double; phase_estimated output double; frequency output double; B input double; Rocof output double
function [amplitude, phase_estimated,frequency,Rocof] = CSTFM(y,f1,B)
pstima = pinv(B)*y;%(101:400);
ph_0 = pstima(3,:)+conj(pstima(4,:));
ph_1 = pstima(2,:)+conj(pstima(5,:));
ph_2 = pstima(1,:)+conj(pstima(6,:));

amplitude=abs(ph_0);
phase_estimated= angle(ph_0);

%% 1st order
%der_amp=2*real(ph_1*exp(-1j*phase_estimated)); % non utilizzata per il momento
der_phase=imag(ph_1*exp(-1j*phase_estimated))/amplitude;
frequency=f1+(der_phase/(2*pi));
der_amp=2*real(ph_1.*exp(-1j*phase_estimated));
%% 2nd order
der2_phase=(imag(ph_2.*exp(-1j*phase_estimated)) ...
        - 2*der_amp.*der_phase)./(amplitude); % seconda derivata fase
Rocof= der2_phase/(2*pi); % stima rocof, Hz/s
end

== matlab function P-class PMU cs-TFM/Subsystem/MATLAB Function2 ==
  data: v input double; D_funda input double; Supp_ord output double
function Supp_ord   = RunOMP_IMEKO_3cycles(v,D_funda)
% index_tot=[23 34 45 56 83 89 94 100];
r_funda=D_funda*(v);
[maxVal, maxPos] = max(r_funda);
Supp_ord=zeros(1,1);
Supp_ord(1) = maxPos(1) + 29;%maxPos(1)+49; %% +50-1 due to look up table 0 based
% v = abs(v)-abs(maxVal*transpose(dft_rec(maxPos,:)));
% r_inter=D_inter*(v);
% [ma_inter,ab_inter]=max(r_inter);
% if abs(ma_inter)>=0.08*abs(maxVal)
%     Supp_ord(2)=index_tot(ab_inter)-1; % due to the zeroth based look-up table
% else
%     Supp_ord(2)=0;
% end
end

== matlab function P-class PMU cs-TFM/Subsystem/MATLAB Function4 ==
  data: matrix_funda input double; matrix_har2 input double; matrix_har3 input double; matrix_out output double
function matrix_out =matrixTaylorFourier_ih2(matrix_funda, matrix_har2, matrix_har3)
% function [matrix]=matrixTaylorFourier_ih(f1, fs, N, orders, harmonics)
% in: f1 - freq di osservazione
%     fs - freq di campionamento
%     N - numero di campioni
%     orders - vettore ordini dell'espansione di Taylor delle harmonics
%     harmonics - vector of harmonic/interharmonic indexes
%     without_sampling - flag to use Ts in the matrix columns
% out: matrix matrice di TaylorFourier
fs=5e3;
harmonics = 1;
if harmonics >5
    Ts=1/fs;
    numcoH =12;
    N=300;
    order=2;
    matrix = complex(zeros(N, numcoH/2));
    Nh=N/2;
    for i=0:N-1
        n = i - Nh;
        nc = 0;
        h=harmonics;
        facts = factorial(order:-1:0);
        if (h==0) % continuous component
            nc = order + 1;
            matrix(i+1,1:nc) = ((n*Ts).^(order:-1:0))./facts;
        else
            e = exp(1j*n*h*2*pi/fs);
            matrix(i+1,nc+1:nc+2*order+2) = [(((n*Ts).^(order:-1:0)).*e)./facts, (((n*Ts).^(0:1:order)).*e')./fliplr(facts)];
            nc = nc+2*order+2;
        end
    end
    matrix_out=[matrix_funda matrix_har2 matrix_har3 matrix];
else
    matrix_out=[matrix_funda matrix_har2 matrix_har3 zeros(300,6)];
%     matrix_out=[matrix_funda zeros(300,6)];
end
end
